simulink library "NeuroMuscularLibrary"  (R2019a)
settings: Solver=ode45  StartTime=0.0  StopTime=10.0  RelTol=1e-3  EnableMultiTasking=on
undefined symbols (not defined in the file): a2loptHAB, a2loptHAD, a2loptHAMsw, a2loptRFsw, ankle_height, aRefHAB, aRefHAD, aRefHAMsw, aRefRFsw, c, c_jointstop, deltaLegAngleThr, DeltaThRef, eref, Fmax, FmaxGLU, footBallToAnkleDist, footBallToCGDist, footBallToCGDist_y, footBallToHeelDist, footCenterlineToBall, footCenterlineToHeel, footInertia, footLength, footMass, FT, FT_GLU, GainDphiHATGLUst, GainDphiHATHABst, GainDphiHATHADst, GainDphiHATHFLst, GainFGASst, GainFGLUst, GainFHABst, GainFHAMst, GainFSOLst, GainFSOLTAst, GainFVASst, GainLBFSHst, GainLBFSHVASst, GainLGLUsw, GainLHABsw, GainLHADsw, GainLHAMGLUsw, GainLHAMsw, GainLRFHFLsw, GainLTAst, GainLTAsw, GainLVASsw, GainPhiHATGLUst, GainPhiHATHABst, GainPhiHATHADst, GainPhiHATHFLst, GainSGLUcHFLst, GainSGLUHAMst, GainSHABcHABst, GainSHADcHADst, GainSHAMBFSHsw, GainSHAMcHFLst, GainSHAMGASsw ... (+175)
libraries: sm_lib x54, $bdroot x45, nesl_utility x39, simulink x24, simulink_extras x6, vrlib x5, dspsigops x4
(part 2 of 5)

== system NeuroMuscularLibrary/Ground Contact Model 3D ==
  note: 3D Ground Interaction Model
  Env : Inport
  " contact sensor" : simulink/Logic and Bit Operations/Compare To Zero  relop=<=  OutDataTypeStr=boolean
  3D Contact : Subsystem
  Demux : Demux  Outputs=3
  Demux2 : Demux  Outputs=6
  Demux3 : Demux  Outputs=[1 3 3]
  External Force and Torque : sm_lib/Forces and Torques/External Force and Torque  ForceResolutionFrame=World  EnableForceX=on  EnableForceY=on  EnableForceZ=on  EnableForce=off  TorqueResolutionFrame=AttachedFrame  EnableTorqueX=off  EnableTorqueY=off  EnableTorqueZ=off  EnableTorque=off
  Mux1 : Mux  Inputs=3
  Mux2 : Mux  Inputs=3
  Position Velocity Sensor : $bdroot/Position Velocity Sensor  SystemSampleTime=-1
  Simulink-PS Converter : nesl_utility/Simulink-PS Converter  PhysicalDomain=network_engine_domain  SubClassName=ps_input  LeftPortType=input  RightPortType=output  PseudoPeriodic=off  Frequencies=[]  NoiseDistribution=none  NoiseParameters=[]  Unit=1  AffineConversion=off  FilteringAndDerivatives=zero  SimscapeFilterOrder=1  InputFilterTimeConstant=0.001  UdotUserProvided=1
  Simulink-PS Converter1 : nesl_utility/Simulink-PS Converter  PhysicalDomain=network_engine_domain  SubClassName=ps_input  LeftPortType=input  RightPortType=output  PseudoPeriodic=off  Frequencies=[]  NoiseDistribution=none  NoiseParameters=[]  Unit=1  AffineConversion=off  FilteringAndDerivatives=zero  SimscapeFilterOrder=1  InputFilterTimeConstant=0.001  UdotUserProvided=1
  Simulink-PS Converter2 : nesl_utility/Simulink-PS Converter  PhysicalDomain=network_engine_domain  SubClassName=ps_input  LeftPortType=input  RightPortType=output  PseudoPeriodic=off  Frequencies=[]  NoiseDistribution=none  NoiseParameters=[]  Unit=1  AffineConversion=off  FilteringAndDerivatives=provide  SimscapeFilterOrder=1  InputFilterTimeConstant=0.001  UdotUserProvided=0
  Sum2 : Sum  Inputs=-+|
  Sum3 : Sum
  Foot : PMIOPort  Side=Left
  Contact? : Outport  VectorParamsAs1DForOutWhenUnconnected=on
  GRF [N N N] : Outport  Port=2  VectorParamsAs1DForOutWhenUnconnected=on
  wires:
  Demux2/1 -> Mux1/1  "x"
  Demux/1 -> Simulink-PS Converter/1
  Mux2/1 -> 3D Contact/4(vVec [m/s m/s m/s])
  Demux2/5 -> Mux2/2  "dy"
  " contact sensor"/1 -> Contact?/1, 3D Contact/Enable
  3D Contact/2(FtVec [N N N]) -> Sum3/2
  Demux/2 -> Simulink-PS Converter1/1
  Demux2/4 -> Mux2/1  "dx"
  3D Contact/1(FnVec [N N N]) -> Sum3/1
  Demux2/2 -> Mux1/2  "y"
  Sum2/1 -> " contact sensor"/1
  Sum3/1 -> Demux/1, GRF [N N N]/1
  Demux2/3 -> Sum2/2, Mux1/3  "z"
  Demux2/6 -> Mux2/3  "dz"
  Demux/3 -> Simulink-PS Converter2/1
  Demux3/3 -> 3D Contact/2(nVec [m m m])  "Normal Vector"
  Mux1/1 -> 3D Contact/3(pVec [m m m])  "pos"
  Demux3/1 -> Sum2/1  "Ground Height"
  Position Velocity Sensor/1 -> Demux2/1
  Env/1 -> Demux3/1
  Demux3/2 -> 3D Contact/1(RefPt [m m m])  "Reference Point"
  connections:
  External Force and Torque/RConn1 -- Foot/RConn1 -- Position Velocity Sensor/LConn1
  External Force and Torque/LConn1 -- Simulink-PS Converter/RConn1
  External Force and Torque/LConn2 -- Simulink-PS Converter1/RConn1
  Simulink-PS Converter2/RConn1 -- External Force and Torque/LConn3

== system NeuroMuscularLibrary/Ground Height Lookup 3D ==
  LHeel+ : Inport
  LHeel- : Inport  Port=2
  LBall+ : Inport  Port=3
  LBall- : Inport  Port=4
  RHeel+ : Inport  Port=5
  RHeel- : Inport  Port=6
  RBall+ : Inport  Port=7
  RBall- : Inport  Port=8
  HATCG : Inport  Port=9
  Env Lookup{,1..8} (9 alike) : $bdroot/Env Lookup  SystemSampleTime=-1  Latency=0  AutoFrameSizeCalculation=off
  Selector : Selector  InputPortWidth=7  IndexOptions=Index vector (dialog)  Indices=[1]  OutputSizes=1
  Selector1 : Selector  InputPortWidth=6  IndexOptions=Index vector (dialog)  Indices=[1 2 3]  OutputSizes=1
  LHeel+Env : Outport  OutputWhenDisabled=reset  InitialOutput=0  VectorParamsAs1DForOutWhenUnconnected=on
  LHeel-Env : Outport  Port=2  OutputWhenDisabled=reset  InitialOutput=0  VectorParamsAs1DForOutWhenUnconnected=on
  LBallEnv : Outport  Port=3  OutputWhenDisabled=reset  InitialOutput=0  VectorParamsAs1DForOutWhenUnconnected=on
  LBall-Env : Outport  Port=4  OutputWhenDisabled=reset  InitialOutput=0  VectorParamsAs1DForOutWhenUnconnected=on
  RHeel+Env : Outport  Port=5  OutputWhenDisabled=reset  InitialOutput=0  VectorParamsAs1DForOutWhenUnconnected=on
  RHeel-Env : Outport  Port=6  OutputWhenDisabled=reset  InitialOutput=0  VectorParamsAs1DForOutWhenUnconnected=on
  RBall+Env : Outport  Port=7  OutputWhenDisabled=reset  InitialOutput=0  VectorParamsAs1DForOutWhenUnconnected=on
  RBall-Env : Outport  Port=8  OutputWhenDisabled=reset  InitialOutput=0  VectorParamsAs1DForOutWhenUnconnected=on
  "HATGroundz " : Outport  Port=9  OutputWhenDisabled=reset  InitialOutput=0  VectorParamsAs1DForOutWhenUnconnected=on
  wires:
  Selector/1 -> "HATGroundz "/1
  Env Lookup8/1 -> Selector/1
  HATCG/1 -> Selector1/1
  Env Lookup6/1 -> RBall+Env/1
  Env Lookup4/1 -> RHeel+Env/1
  RBall+/1 -> Env Lookup6/1
  RHeel+/1 -> Env Lookup4/1
  Env Lookup2/1 -> LBallEnv/1
  LBall+/1 -> Env Lookup2/1
  Env Lookup/1 -> LHeel+Env/1
  LHeel+/1 -> Env Lookup/1
  LHeel-/1 -> Env Lookup1/1
  Env Lookup1/1 -> LHeel-Env/1
  LBall-/1 -> Env Lookup3/1
  Env Lookup3/1 -> LBall-Env/1
  RHeel-/1 -> Env Lookup5/1
  Env Lookup5/1 -> RHeel-Env/1
  RBall-/1 -> Env Lookup7/1
  Env Lookup7/1 -> RBall-Env/1
  Selector1/1 -> Env Lookup8/1

== system NeuroMuscularLibrary/HAB Link ==
  note: HAB Attachment
  Hip roll angle [rad] : Inport
  Constant : Constant  Value=lslackHAB+loptHAB
  Constant1 : Constant  Value=rHAB
  Constant2 : Constant  Value=phirefHAB
  Gain2 : Gain  Gain=rhoHAB
  Product : Product  RndMeth=Zero
  Sum2 : Sum  Inputs=|+-
  Sum5 : Sum  Inputs=|+-
  lmtu [m] : Outport  VectorParamsAs1DForOutWhenUnconnected=on
  lever [m] : Outport  Port=2  VectorParamsAs1DForOutWhenUnconnected=on
  wires:
  Gain2/1 -> Sum5/2
  Constant1/1 -> lever [m]/1, Product/2
  Sum2/1 -> Product/1
  Constant2/1 -> Sum2/2
  Hip roll angle [rad]/1 -> Sum2/1
  Product/1 -> Gain2/1
  Sum5/1 -> lmtu [m]/1
  Constant/1 -> Sum5/1

== system NeuroMuscularLibrary/HAD Link ==
  note: HAD Attachment
  hip roll angle [rad] : Inport
  Constant : Constant  Value=lslackHAD+loptHAD
  Constant1 : Constant  Value=rHAD
  Constant2 : Constant  Value=phirefHAD
  Gain2 : Gain  Gain=rhoHAD
  Product : Product  RndMeth=Zero
  Sum2 : Sum  Inputs=|+-
  Sum5 : Sum  Inputs=|++
  lmtu [m] : Outport  VectorParamsAs1DForOutWhenUnconnected=on
  lever [m] : Outport  Port=2  VectorParamsAs1DForOutWhenUnconnected=on
  wires:
  Constant/1 -> Sum5/1
  Sum5/1 -> lmtu [m]/1
  Product/1 -> Gain2/1
  hip roll angle [rad]/1 -> Sum2/1
  Constant2/1 -> Sum2/2
  Sum2/1 -> Product/1
  Constant1/1 -> Product/2, lever [m]/1
  Gain2/1 -> Sum5/2

== system NeuroMuscularLibrary/HAM Link ==
  note: HAM Attachment
  hip angle : Inport
  knee angle : Inport  Port=2
  Constant1 : Constant  Value=rHAMk
  Constant10 : Constant  Value=phirefHAMh
  Constant2 : Constant  Value=phirefHAMk
  Constant8 : Constant  Value=rHAMh
  Constant9 : Constant  Value=lslackHAM+loptHAM
  Gain1 : Gain  Gain=rhoHAMh
  Gain5 : Gain  Gain=rhoHAMk
  Product1 : Product  RndMeth=Zero
  Product2 : Product  RndMeth=Zero
  Sum1 : Sum  Inputs=|+-
  Sum2 : Sum  Inputs=|+-
  Sum3 : Sum  Inputs=-+-
  lmtu [m] : Outport  VectorParamsAs1DForOutWhenUnconnected=on
  hip lever [m] : Outport  Port=2  VectorParamsAs1DForOutWhenUnconnected=on
  knee lever [m] : Outport  Port=3  VectorParamsAs1DForOutWhenUnconnected=on
  wires:
  Sum1/1 -> Product2/1
  Constant1/1 -> knee lever [m]/1, Product2/2
  Product1/1 -> Gain1/1
  Constant2/1 -> Sum1/2
  Sum3/1 -> lmtu [m]/1
  Gain1/1 -> Sum3/1
  Constant10/1 -> Sum2/2
  Constant8/1 -> hip lever [m]/1, Product1/2
  Constant9/1 -> Sum3/2
  Gain5/1 -> Sum3/3
  Sum2/1 -> Product1/1
  hip angle/1 -> Sum2/1
  knee angle/1 -> Sum1/1
  Product2/1 -> Gain5/1

== system NeuroMuscularLibrary/HAM amp Link ==
  note: HAM Attachment
  hip angle : Inport
  Constant10 : Constant  Value=phirefHAMh
  Constant8 : Constant  Value=rHAMh
  Constant9 : Constant  Value=lslackHAMamp+loptHAMamp
  Gain1 : Gain  Gain=rhoHAMh
  Product1 : Product  RndMeth=Zero
  Sum2 : Sum  Inputs=|+-
  Sum3 : Sum  Inputs=-+
  lmtu [m] : Outport  VectorParamsAs1DForOutWhenUnconnected=on
  hip lever [m] : Outport  Port=2  VectorParamsAs1DForOutWhenUnconnected=on
  wires:
  hip angle/1 -> Sum2/1
  Sum2/1 -> Product1/1
  Constant9/1 -> Sum3/2
  Constant8/1 -> Product1/2, hip lever [m]/1
  Constant10/1 -> Sum2/2
  Gain1/1 -> Sum3/1
  Sum3/1 -> lmtu [m]/1
  Product1/1 -> Gain1/1

== system NeuroMuscularLibrary/HATs ==
  Brick Solid : sm_lib/Body Elements/Solid  InertiaType=CalculateFromGeometry  Mass=0  MassUnits=kg  CenterOfMass=[0 0 0]  CenterOfMassUnits=m  MomentsOfInertia=[1 1 1]  MomentsOfInertiaUnits=kg*m^2  ProductsOfInertia=[0 0 0]  ProductsOfInertiaUnits=kg*m^2  BasedOnType=Mass  Density=0  DensityUnits=kg/m^3  DoExposeReferenceFrame=on  SerializedFrames=<Frames/>  GraphicType=FromGeometry  MarkerShape=Sphere  MarkerSize=10  GraphicVisPropType=SimpleVisualProperties  GraphicDiffuseColor=[0.5 0.5 0.5]  GraphicSpecularColor=[0.5 0.5 0.5 1.0]  GraphicAmbientColor=[0.15 0.15 0.15 1.0]  GraphicEmissiveColor=[0.0 0.0 0.0 1.0]  GraphicShininess=75  GraphicOpacity=1.0  GeometryShape=Brick  RectangleSize=[1 1]  RectangleSizeUnits=m  BrickDimensions=[hatLength hatThickness hatWidth]  BrickDimensionUnits=m  CylinderRadius=1  CylinderRadiusUnits=m  CylinderLength=1  CylinderLengthUnits=m  SphereRadius=1  SphereRadiusUnits=m  EllipsoidRadii=[1 1 1]  EllipsoidRadiiUnits=m  ExtrusionCrossSection=[1 1; -1 1; -1 -1; 1 -1]  ExtrusionCrossSectionUnits=m  ExtrusionLength=1  ExtrusionLengthUnits=m  PolygonNumSides=3  PolygonOuterRadius=1  PolygonOuterRadiusUnits=m  ExtGeomFileType=STEP  ExtGeomFileUnits=m  RevolutionCrossSection=[1 1; 1 -1; 2 -1; 2 1]  RevolutionCrossSectionUnits=m  RevolutionExtent=Full  RevolutionAngle=180  RevolutionAngleUnits=deg
  Inertia : sm_lib/Body Elements/Inertia  InertiaType=Custom  Mass=hatMass  MassUnits=kg  CenterOfMass=[0 0 0]  CenterOfMassUnits=m  MomentsOfInertia=hatInertia  MomentsOfInertiaUnits=kg*m^2  ProductsOfInertia=[0 0 0]  ProductsOfInertiaUnits=kg*m^2  GraphicType=None  MarkerShape=Inertia  MarkerSize=20  GraphicVisPropType=SimpleVisualProperties  GraphicDiffuseColor=[0.5 0.5 0.5]  GraphicSpecularColor=[0.5 0.5 0.5 1.0]  GraphicAmbientColor=[0.15 0.15 0.15 1.0]  GraphicEmissiveColor=[0.0 0.0 0.0 1.0]  GraphicShininess=75  GraphicOpacity=1.0
  Rigid Transform : sm_lib/Frames and Transforms/Rigid Transform  TranslationMethod=None  TranslationStandardOffset=0  TranslationLengthUnit=m  TranslationStandardAxis=+Z  TranslationCartesianOffset=[0 0 0]  TranslationROffset=0  TranslationROffsetUnits=m  TranslationZOffset=0  TranslationZOffsetUnits=m  TranslationThetaOffset=0  TranslationThetaOffsetUnits=deg  RotationMethod=AlignedAxes  RotationAngleUnits=deg  RotationStandardAxis=+Z  RotationAngle=0.0  RotationArbitraryAxis=[0 0 1]  FollAlignAxisA=+X  BaseAlignAxisA=-Y  FollAlignAxisB=+Z  BaseAlignAxisB=+X  RotationSequenceAxes=FollowerAxes  RotationSequence=XYX  RotationSequenceAngles=[0 0 0]  RotationSequenceAnglesUnits=deg  RotationMatrix=[1 0 0; 0 1 0; 0 0 1]
  To CG : sm_lib/Frames and Transforms/Rigid Transform  TranslationMethod=Cartesian  TranslationStandardOffset=0  TranslationLengthUnit=m  TranslationStandardAxis=+Z  TranslationCartesianOffset=[hatLeftHipToCG 0 hatLeftHipToCenterDistWidth]  TranslationROffset=0  TranslationROffsetUnits=m  TranslationZOffset=0  TranslationZOffsetUnits=m  TranslationThetaOffset=0  TranslationThetaOffsetUnits=deg  RotationMethod=None  RotationAngleUnits=deg  RotationStandardAxis=+Z  RotationAngle=0.0  RotationArbitraryAxis=[0 0 1]  FollAlignAxisA=+X  BaseAlignAxisA=-Y  FollAlignAxisB=+Z  BaseAlignAxisB=+X  RotationSequenceAxes=FollowerAxes  RotationSequence=XYX  RotationSequenceAngles=[0 0 0]  RotationSequenceAnglesUnits=deg  RotationMatrix=[1 0 0; 0 1 0; 0 0 1]
  To center : sm_lib/Frames and Transforms/Rigid Transform  TranslationMethod=Cartesian  TranslationStandardOffset=0  TranslationLengthUnit=m  TranslationStandardAxis=+Z  TranslationCartesianOffset=[hatLength/2 0 hatLeftHipToCenterDistWidth]  TranslationROffset=0  TranslationROffsetUnits=m  TranslationZOffset=0  TranslationZOffsetUnits=m  TranslationThetaOffset=0  TranslationThetaOffsetUnits=deg  RotationMethod=None  RotationAngleUnits=deg  RotationStandardAxis=+Z  RotationAngle=0.0  RotationArbitraryAxis=[0 0 1]  FollAlignAxisA=+Z  BaseAlignAxisA=-X  FollAlignAxisB=+Y  BaseAlignAxisB=+Y  RotationSequenceAxes=FollowerAxes  RotationSequence=XYX  RotationSequenceAngles=[0 0 0]  RotationSequenceAnglesUnits=deg  RotationMatrix=[1 0 0; 0 1 0; 0 0 1]
  To right hip : sm_lib/Frames and Transforms/Rigid Transform  TranslationMethod=Cartesian  TranslationStandardOffset=0  TranslationLengthUnit=m  TranslationStandardAxis=+Z  TranslationCartesianOffset=[-2*hatLeftHipToCenterDistWidth 0 0]  TranslationROffset=0  TranslationROffsetUnits=m  TranslationZOffset=0  TranslationZOffsetUnits=m  TranslationThetaOffset=0  TranslationThetaOffsetUnits=deg  RotationMethod=AlignedAxes  RotationAngleUnits=deg  RotationStandardAxis=+Z  RotationAngle=0.0  RotationArbitraryAxis=[0 0 1]  FollAlignAxisA=+X  BaseAlignAxisA=-Z  FollAlignAxisB=+Y  BaseAlignAxisB=+Y  RotationSequenceAxes=FollowerAxes  RotationSequence=XYX  RotationSequenceAngles=[0 0 0]  RotationSequenceAnglesUnits=deg  RotationMatrix=[1 0 0; 0 1 0; 0 0 1]
  To top : sm_lib/Frames and Transforms/Rigid Transform  TranslationMethod=Cartesian  TranslationStandardOffset=0  TranslationLengthUnit=m  TranslationStandardAxis=+Z  TranslationCartesianOffset=[hatLength 0 hatLeftHipToCenterDistWidth]  TranslationROffset=0  TranslationROffsetUnits=m  TranslationZOffset=0  TranslationZOffsetUnits=m  TranslationThetaOffset=0  TranslationThetaOffsetUnits=deg  RotationMethod=None  RotationAngleUnits=deg  RotationStandardAxis=+Z  RotationAngle=0.0  RotationArbitraryAxis=[0 0 1]  FollAlignAxisA=+X  BaseAlignAxisA=+Y  FollAlignAxisB=+Y  BaseAlignAxisB=+Z  RotationSequenceAxes=FollowerAxes  RotationSequence=XYX  RotationSequenceAngles=[0 0 0]  RotationSequenceAnglesUnits=deg  RotationMatrix=[1 0 0; 0 1 0; 0 0 1]
  "X-medial,  Y-back Z-up, to X-up, Y-back, Z lateral" : sm_lib/Frames and Transforms/Rigid Transform  TranslationMethod=None  TranslationStandardOffset=0  TranslationLengthUnit=m  TranslationStandardAxis=+Z  TranslationCartesianOffset=[0 0 0]  TranslationROffset=0  TranslationROffsetUnits=m  TranslationZOffset=0  TranslationZOffsetUnits=m  TranslationThetaOffset=0  TranslationThetaOffsetUnits=deg  RotationMethod=AlignedAxes  RotationAngleUnits=deg  RotationStandardAxis=+Z  RotationAngle=0.0  RotationArbitraryAxis=[0 0 1]  FollAlignAxisA=+X  BaseAlignAxisA=-Z  FollAlignAxisB=+Y  BaseAlignAxisB=+Y  RotationSequenceAxes=FollowerAxes  RotationSequence=XYX  RotationSequenceAngles=[0 0 0]  RotationSequenceAnglesUnits=deg  RotationMatrix=[1 0 0; 0 1 0; 0 0 1]
  Left hip : PMIOPort  Side=Left
  Right hip : PMIOPort  Port=2  Side=Left
  CG : PMIOPort  Port=3  Side=Right
  Top : PMIOPort  Port=4  Side=Right
  connections:
  To center/LConn1 -- To top/LConn1 -- To right hip/RConn1 -- To CG/LConn1 -- "X-medial,  Y-back Z-up, to X-up, Y-back, Z lateral"/RConn1
  Brick Solid/RConn1 -- To center/RConn1
  To right hip/LConn1 -- Right hip/RConn1
  Left hip/RConn1 -- "X-medial,  Y-back Z-up, to X-up, Y-back, Z lateral"/LConn1
  CG/RConn1 -- Rigid Transform/RConn1 -- Inertia/RConn1
  To CG/RConn1 -- Rigid Transform/LConn1
  Top/RConn1 -- To top/RConn1

== system NeuroMuscularLibrary/HFL Link ==
  note: HFL Attachment
  hip angle [rad] : Inport
  Constant : Constant  Value=lslackHFL+loptHFL
  Constant1 : Constant  Value=rHFL
  Constant2 : Constant  Value=phirefHFL
  Gain2 : Gain  Gain=rhoHFL
  Product : Product  RndMeth=Zero
  Sum2 : Sum  Inputs=|+-
  Sum5 : Sum  Inputs=|++
  lmtu [m] : Outport  VectorParamsAs1DForOutWhenUnconnected=on
  lever [m] : Outport  Port=2  VectorParamsAs1DForOutWhenUnconnected=on
  wires:
  Constant/1 -> Sum5/1
  Sum5/1 -> lmtu [m]/1
  Product/1 -> Gain2/1
  Constant2/1 -> Sum2/2
  Sum2/1 -> Product/1
  Constant1/1 -> Product/2, lever [m]/1
  Gain2/1 -> Sum5/2
  hip angle [rad]/1 -> Sum2/1

== system NeuroMuscularLibrary/Hard Stops ==
  Muscle Torques : Inport
  phiANDdphiHip : Inport  Port=2
  phiANDdphiKnee : Inport  Port=3
  phiANDdphiAnkle : Inport  Port=4
  Muscle Torques R : Inport  Port=5
  phiANDdphiHipR : Inport  Port=6
  Add : Sum
  Add1 : Sum
  Ankle Joint Limit : $bdroot/Overextension//Overflexion Joint Limit  phiUpLimit=phiAnkleUpLimit  phiLowLimit=phiAnkleLowLimit
  Demux{,1..3} (4 alike) : Demux  Outputs=2
  Hip Overextension Joint Limit : $bdroot/Overextension Joint Limit  phiUpLimit=phiHipUpLimit  ext=1
  Hip roll Joint Limit : Subsystem  mask(Overextension/Overflexion Joint Limit){phiUpLimit=phiHipAbdUpLimit, phiLowLimit=phiHipAbdLowLimit}
      mask prompts: phiUpLimit "Upper Limit [rad]"; phiLowLimit "Lower Limit [rad]"
      mask help:
      | This block implents a hard joint limit that will prevent the joint from overextending past the specified upper limit and overflexing below the lower limit.
      |
      | Used for the Ankle Joint.
  Knee Overextension Joint Limit : $bdroot/Overextension Joint Limit  phiUpLimit=phiKneeUpLimit  ext=-1
  Mux : Mux  Inputs=3
  Net Torque : Outport  VectorParamsAs1DForOutWhenUnconnected=on
  Hip Stop Torque : Outport  Port=2  VectorParamsAs1DForOutWhenUnconnected=on
  Knee Stop Torque : Outport  Port=3  VectorParamsAs1DForOutWhenUnconnected=on
  Ankle Stop Torque : Outport  Port=4  VectorParamsAs1DForOutWhenUnconnected=on
  Net Torque R : Outport  Port=5  VectorParamsAs1DForOutWhenUnconnected=on
  Hip R Stop Torque : Outport  Port=6  VectorParamsAs1DForOutWhenUnconnected=on
  wires:
  Knee Overextension Joint Limit/1 -> Knee Stop Torque/1, Mux/2
  Muscle Torques/1 -> Add/1
  Mux/1 -> Add/2
  Ankle Joint Limit/1 -> Ankle Stop Torque/1, Mux/3
  Demux/2 -> Knee Overextension Joint Limit/2
  Demux/1 -> Knee Overextension Joint Limit/1
  Demux1/1 -> Hip Overextension Joint Limit/1
  Demux1/2 -> Hip Overextension Joint Limit/2
  Demux2/1 -> Ankle Joint Limit/1
  Demux2/2 -> Ankle Joint Limit/2
  phiANDdphiKnee/1 -> Demux/1
  Hip Overextension Joint Limit/1 -> Hip Stop Torque/1, Mux/1
  phiANDdphiHip/1 -> Demux1/1
  phiANDdphiAnkle/1 -> Demux2/1
  Add/1 -> Net Torque/1
  Demux3/2 -> Hip roll Joint Limit/2(dphi [rad/s])
  Demux3/1 -> Hip roll Joint Limit/1(phi [rad])
  phiANDdphiHipR/1 -> Demux3/1
  Add1/1 -> Net Torque R/1
  Hip roll Joint Limit/1(M_stop [Nm]) -> Hip R Stop Torque/1, Add1/2
  Muscle Torques R/1 -> Add1/1

== system NeuroMuscularLibrary/Hill Muscle ==
  note: Excitation Contraction Coupling
  note: Muscle-Tendon Dynamics
  STIM : Inport
  lmtc [m] : Inport  Port=2
  1 : Product  Inputs=**  SaturateOnIntegerOverflow=on  InputSameDT=on  OutDataTypeStr=Inherit: Same as first input
  1/lslack : Gain  Gain=1/lslack  SaturateOnIntegerOverflow=on  OutDataTypeStr=Inherit: Same as input  ParamDataTypeStr=Inherit: Same as input
  Add : Sum  Inputs=+-
  BE force-length relation : Subsystem
  CE force-length relation : Subsystem
  CE inverse force-velocity relation : Subsystem
  Constant : Constant  Value=lslack
  ECC TransferFcn : simulink_extras/Additional Linear/Transfer Fcn (with initial outputs)  N=[1]  D="[tau  1]"  Y0=preA  U0=0
      settings: AttributesFormatString=pre-activation: %<Y0>
  Fmax : Gain  Gain=Fmax  SaturateOnIntegerOverflow=on  OutDataTypeStr=Inherit: Same as input  ParamDataTypeStr=Inherit: Same as input
  Fv = Fse / (A*Fce) : Product  Inputs=*/  SaturateOnIntegerOverflow=on  InputSameDT=on  OutDataTypeStr=Inherit: Same as first input
  Integrator : Integrator  InitialConditionSource=external  LowerSaturationLimit=0.05
  PE force-length relation : Subsystem
  SE force-length relation : Subsystem
  Sum : Sum  Inputs=|+-  SaturateOnIntegerOverflow=on  InputSameDT=on  OutDataTypeStr=Inherit: Same as first input
  Sum2 : Sum  Inputs=|-+  SaturateOnIntegerOverflow=on  InputSameDT=on  OutDataTypeStr=Inherit: Same as first input
  Sum3 : Sum  SaturateOnIntegerOverflow=on  InputSameDT=on  OutDataTypeStr=Inherit: Same as first input
  Sum4 : Sum  SaturateOnIntegerOverflow=on  InputSameDT=on  OutDataTypeStr=Inherit: Same as first input
  lce/lopt : Gain  Gain=1/lopt  SaturateOnIntegerOverflow=on  OutDataTypeStr=Inherit: Same as input  ParamDataTypeStr=Inherit: Same as input
  lce/lopt1 : Gain  Gain=1/lopt  SaturateOnIntegerOverflow=on  OutDataTypeStr=Inherit: Same as input  ParamDataTypeStr=Inherit: Same as input
  lopt : Gain  Gain=lopt  SaturateOnIntegerOverflow=on  OutDataTypeStr=Inherit: Same as input  ParamDataTypeStr=Inherit: Same as input
  vmax : Gain  Gain=vmax  SaturateOnIntegerOverflow=on  OutDataTypeStr=Inherit: Same as input  ParamDataTypeStr=Inherit: Same as input
  Fmtc : Outport  InitialOutput=0  VectorParamsAs1DForOutWhenUnconnected=on
  Lce [lopt] : Outport  Port=2  InitialOutput=0  VectorParamsAs1DForOutWhenUnconnected=on
  Vce [lopt] : Outport  Port=3  InitialOutput=0  VectorParamsAs1DForOutWhenUnconnected=on
  Lse : Outport  Port=4  InitialOutput=0  VectorParamsAs1DForOutWhenUnconnected=on
  A : Outport  Port=5  InitialOutput=0  VectorParamsAs1DForOutWhenUnconnected=on
  fce : Outport  Port=6  VectorParamsAs1DForOutWhenUnconnected=on
  wires:
  ECC TransferFcn/1 -> 1/2, A/1
  STIM/1 -> ECC TransferFcn/1
  CE inverse force-velocity relation/1(v[vmax]) -> vmax/1
  Sum3/1 -> Fv = Fse / (A*Fce)/2
  BE force-length relation/1(fbe [Fmax]) -> Sum4/2
  1/1 -> Sum3/2
  PE force-length relation/1(fpe [Fmax]) -> Sum3/1, Add/2
  Sum4/1 -> Add/1, Fv = Fse / (A*Fce)/1  "fse+fbe"
  CE force-length relation/1(fce [Fmax]) -> 1/1  "f_l"
  Constant/1 -> Sum2/1
  Sum2/1 -> Integrator/2
  SE force-length relation/1(fse [Fmax]) -> Sum4/1, Fmax/1
  1/lslack/1 -> SE force-length relation/1(lse [lslack])
  Fmax/1 -> Fmtc/1  "Fmtc"
  lmtc [m]/1 -> Sum/1, Sum2/2  "lmtc"
  vmax/1 -> lopt/1, Vce [lopt]/1  "vce"
  Fv = Fse / (A*Fce)/1 -> CE inverse force-velocity relation/1(Fv[Fmax])  "fv"
  lce/lopt/1 -> PE force-length relation/1(lce [lopt]), BE force-length relation/1(lce [lopt]), CE force-length relation/1(lce [lopt])
  Sum/1 -> Lse/1, 1/lslack/1  "lse"
  Integrator/1 -> lce/lopt1/1, lce/lopt/1, Sum/2  "lce"
  Add/1 -> fce/1
  lce/lopt1/1 -> Lce [lopt]/1
  lopt/1 -> Integrator/1  "vce"

== system NeuroMuscularLibrary/Leg Angle//Length ==
  Constant : Constant  Value=pi
  Demux : Demux  Outputs=2
  Mux : Mux  Inputs=3
  Mux1 : Mux  Inputs=3
  PS-Simulink Converter{,1..6} (7 alike) : nesl_utility/PS-Simulink Converter  PhysicalDomain=network_engine_domain  SubClassName=ps_output  LeftPortType=input  RightPortType=output  PseudoPeriodic=off  Frequencies=[]  Unit=m  AffineConversion=off
  Position Sensor : sm_lib/Frames and Transforms/Transform Sensor  MeasurementFrame=World  SenseAngle=off  SenseAxis=off  SenseAngle1=off  SenseAngle2=off  SenseAngle3=off  SenseQ=off  SenseR=off  SenseOmegaX=off  SenseOmegaY=off  SenseOmegaZ=off  SenseOmega1=off  SenseOmega2=off  SenseOmega3=off  SenseQDot=off  SenseRDot=off  SenseAlphaX=off  SenseAlphaY=off  SenseAlphaZ=off  SenseAlpha1=off  SenseAlpha2=off  SenseAlpha3=off  SenseQDDot=off  SenseRDDot=off  SenseX=on  SenseY=on  SenseZ=on  SenseRad=off  SenseAzim=off  SenseDist=off  SenseInc=off  SenseXDot=off  SenseYDot=off  SenseZDot=off  SenseRadDot=off  SenseAzimDot=off  SenseDistDot=off  SenseIncDot=off  SenseXDDot=off  SenseYDDot=off  SenseZDDot=off  SenseRadDDot=off  SenseAzimDDot=off  SenseDistDDot=off  SenseIncDDot=off
  Position Sensor1 : sm_lib/Frames and Transforms/Transform Sensor  MeasurementFrame=World  SenseAngle=off  SenseAxis=off  SenseAngle1=off  SenseAngle2=off  SenseAngle3=off  SenseQ=off  SenseR=off  SenseOmegaX=off  SenseOmegaY=off  SenseOmegaZ=off  SenseOmega1=off  SenseOmega2=off  SenseOmega3=off  SenseQDot=off  SenseRDot=off  SenseAlphaX=off  SenseAlphaY=off  SenseAlphaZ=off  SenseAlpha1=off  SenseAlpha2=off  SenseAlpha3=off  SenseQDDot=off  SenseRDDot=off  SenseX=on  SenseY=on  SenseZ=on  SenseRad=off  SenseAzim=off  SenseDist=off  SenseInc=off  SenseXDot=off  SenseYDot=off  SenseZDot=off  SenseRadDot=off  SenseAzimDot=off  SenseDistDot=off  SenseIncDot=off  SenseXDDot=off  SenseYDDot=off  SenseZDDot=off  SenseRadDDot=off  SenseAzimDDot=off  SenseDistDDot=off  SenseIncDDot=off
  Selector : Selector  InputPortWidth=3  IndexOptions=Index vector (dialog)  Indices=[3 1]  OutputSizes=1
  Subtract : Sum  Inputs=+-
  Sum : Sum  Inputs=|-+
  Transform Sensor : sm_lib/Frames and Transforms/Transform Sensor  MeasurementFrame=World  SenseAngle=off  SenseAxis=off  SenseAngle1=off  SenseAngle2=off  SenseAngle3=off  SenseQ=off  SenseR=off  SenseOmegaX=off  SenseOmegaY=off  SenseOmegaZ=off  SenseOmega1=off  SenseOmega2=off  SenseOmega3=off  SenseQDot=off  SenseRDot=off  SenseAlphaX=off  SenseAlphaY=off  SenseAlphaZ=off  SenseAlpha1=off  SenseAlpha2=off  SenseAlpha3=off  SenseQDDot=off  SenseRDDot=off  SenseX=off  SenseY=off  SenseZ=off  SenseRad=off  SenseAzim=off  SenseDist=on  SenseInc=off  SenseXDot=off  SenseYDot=off  SenseZDot=off  SenseRadDot=off  SenseAzimDot=off  SenseDistDot=off  SenseIncDot=off  SenseXDDot=off  SenseYDDot=off  SenseZDDot=off  SenseRadDDot=off  SenseAzimDDot=off  SenseDistDDot=off  SenseIncDDot=off
  Trigonometric Function : Trigonometry  Operator=atan2  OutputSignalType=real
  World Frame : sm_lib/Frames and Transforms/World Frame
  Hip : PMIOPort  Side=Left
  Ankle : PMIOPort  Port=2  Side=Left
  Leg Angle : Outport  VectorParamsAs1DForOutWhenUnconnected=on
  Leg Length : Outport  Port=2  VectorParamsAs1DForOutWhenUnconnected=on
  wires:
  PS-Simulink Converter6/1 -> Leg Length/1
  PS-Simulink Converter2/1 -> Mux/3
  PS-Simulink Converter/1 -> Mux/1
  PS-Simulink Converter1/1 -> Mux/2
  PS-Simulink Converter5/1 -> Mux1/3
  PS-Simulink Converter3/1 -> Mux1/1
  PS-Simulink Converter4/1 -> Mux1/2
  Mux/1 -> Subtract/1
  Mux1/1 -> Subtract/2
  Trigonometric Function/1 -> Sum/1
  Sum/1 -> Leg Angle/1
  Constant/1 -> Sum/2
  Subtract/1 -> Selector/1
  Selector/1 -> Demux/1
  Demux/1 -> Trigonometric Function/1
  Demux/2 -> Trigonometric Function/2
  connections:
  PS-Simulink Converter6/LConn1 -- Transform Sensor/RConn2
  PS-Simulink Converter2/LConn1 -- Position Sensor/RConn4
  PS-Simulink Converter/LConn1 -- Position Sensor/RConn2
  Transform Sensor/RConn1 -- Hip/RConn1 -- Position Sensor/RConn1
  PS-Simulink Converter1/LConn1 -- Position Sensor/RConn3
  World Frame/RConn1 -- Position Sensor/LConn1 -- Position Sensor1/LConn1
  PS-Simulink Converter4/LConn1 -- Position Sensor1/RConn3
  PS-Simulink Converter5/LConn1 -- Position Sensor1/RConn4
  PS-Simulink Converter3/LConn1 -- Position Sensor1/RConn2
  Transform Sensor/LConn1 -- Ankle/RConn1 -- Position Sensor1/RConn1

== system NeuroMuscularLibrary/Leg Load ==
  dxThigh [m] : Inport
  FB Gain1 : Gain  Gain=1/DeltaThRef  SaturateOnIntegerOverflow=on  OutDataTypeStr=Inherit: Same as input  ParamDataTypeStr=Inherit: Same as input
  Saturation11 : Saturate  UpperLimit=inf  LowerLimit=0  ZeroCross=off
  smooth2 : TransferFcn  Denominator=[0.02 1]
  LLoad [F] : Outport  VectorParamsAs1DForOutWhenUnconnected=on
  wires:
  Saturation11/1 -> FB Gain1/1
  smooth2/1 -> Saturation11/1
  FB Gain1/1 -> LLoad [F]/1
  dxThigh [m]/1 -> smooth2/1

== system NeuroMuscularLibrary/Leg step length//vel calculator ==
  note: Spatial definitions based on Huxham et al. 2006
  Ankle pos : Inport
  Contralateral ankle pos at initial contact : Inport  Port=2
  Simulation time : Inport  Port=3
  Time of contralateral contact : Inport  Port=4
  Prev step number : Inport  Port=5
  Enable : EnablePort
  Add : Sum
  Add2 : Sum  Inputs=-+
  Add3 : Sum  Inputs=+-
  Add4 : Sum  Inputs=+-
  Constant : Constant
  Delay One Step : Delay  DelayLength=1
  Delay One Step1 : Delay  DelayLength=1
  Difference : simulink/Discrete/Difference  ICPrevInput=0.0  OutMin=[]  OutMax=[]  OutDataType=fixdt(1, 16)  OutScaling=2^-10  DoSatur=off
  Divide : Product  Inputs=*/
  Divide1 : Product  Inputs=*/
  Dot Product : DotProduct  InputSameDT=on  OutDataTypeStr=Inherit: Inherit via internal rule
  Norm2 : $bdroot/Norm  SystemSampleTime=-1  Latency=0  AutoFrameSizeCalculation=off
  Product : Product  Inputs=/*
  Selector : Selector  InputPortWidth=3  IndexOptions=Index vector (dialog)  Indices=[1 2]  OutputSizes=1
  Selector1 : Selector  InputPortWidth=3  IndexOptions=Index vector (dialog)  Indices=[1 2]  OutputSizes=1
  Step length : Outport  OutputWhenDisabled=reset  InitialOutput=[0]  VectorParamsAs1DForOutWhenUnconnected=on
  Step time : Outport  Port=2  OutputWhenDisabled=reset  InitialOutput=[0]  VectorParamsAs1DForOutWhenUnconnected=on
  Step avg velocity : Outport  Port=3  OutputWhenDisabled=reset  InitialOutput=[0]  VectorParamsAs1DForOutWhenUnconnected=on
  Stride length : Outport  Port=4  OutputWhenDisabled=reset  InitialOutput=[0]  VectorParamsAs1DForOutWhenUnconnected=on
  Stride time : Outport  Port=5  OutputWhenDisabled=reset  InitialOutput=[0]  VectorParamsAs1DForOutWhenUnconnected=on
  Stride avg velocity : Outport  Port=6  OutputWhenDisabled=reset  InitialOutput=[0]  VectorParamsAs1DForOutWhenUnconnected=on
  Step number : Outport  Port=7  InitialOutput=[0]  VectorParamsAs1DForOutWhenUnconnected=on
  wires:
  Time of contralateral contact/1 -> Add2/1
  Add2/1 -> Step time/1, Divide/2
  Divide/1 -> Step avg velocity/1
  Prev step number/1 -> Delay One Step/1
  Constant/1 -> Add/2
  Add/1 -> Step number/1
  Delay One Step/1 -> Add/1
  Ankle pos/1 -> Selector/1
  Simulation time/1 -> Add2/2, Difference/1
  Add4/1 -> Dot Product/1, Norm2/1
  Delay One Step1/1 -> Add4/2
  Contralateral ankle pos at initial contact/1 -> Selector1/1
  Add3/1 -> Dot Product/2
  Selector/1 -> Add4/1, Delay One Step1/1, Add3/1
  Selector1/1 -> Add3/2
  Norm2/1 -> Product/1, Divide1/1, Stride length/1  "c"
  Difference/1 -> Divide1/2, Stride time/1
  Divide1/1 -> Stride avg velocity/1
  Dot Product/1 -> Product/2
  Product/1 -> Divide/1, Step length/1

== system NeuroMuscularLibrary/Muscle Energy ==
  Dynamics : Inport
  Stimulation : Inport  Port=2
  Muscle Energy Umberger (2003) : $bdroot/Muscle Energy Umberger (2003)  lopt=lopt  FT=FT  Fmax=Fmax  vmax=vmax
  Muscle Energy Umberger (2003) TG : $bdroot/Muscle Energy Umberger (2003) TG  lopt=lopt  FT=FT  Fmax=Fmax
  Muscle Energy Umberger (2010) : $bdroot/Muscle Energy Umberger (2010)  lopt=lopt  FT=FT  Fmax=Fmax  vmax=vmax
  Muscle Energy Wang (2012) : $bdroot/Muscle Energy Wang (2012)  lopt=lopt  FT=FT  Fmax=Fmax
  Mux : Mux
  Power : Outport  VectorParamsAs1DForOutWhenUnconnected=on
  wires:
  Dynamics/1 -> Muscle Energy Umberger (2010)/1, Muscle Energy Umberger (2003) TG/1, Muscle Energy Umberger (2003)/1, Muscle Energy Wang (2012)/1
  Stimulation/1 -> Muscle Energy Umberger (2003)/2, Muscle Energy Umberger (2003) TG/2, Muscle Energy Wang (2012)/2, Muscle Energy Umberger (2010)/2
  Mux/1 -> Power/1
  Muscle Energy Umberger (2003)/1 -> Mux/1
  Muscle Energy Umberger (2003) TG/1 -> Mux/2
  Muscle Energy Umberger (2010)/1 -> Mux/3
  Muscle Energy Wang (2012)/1 -> Mux/4

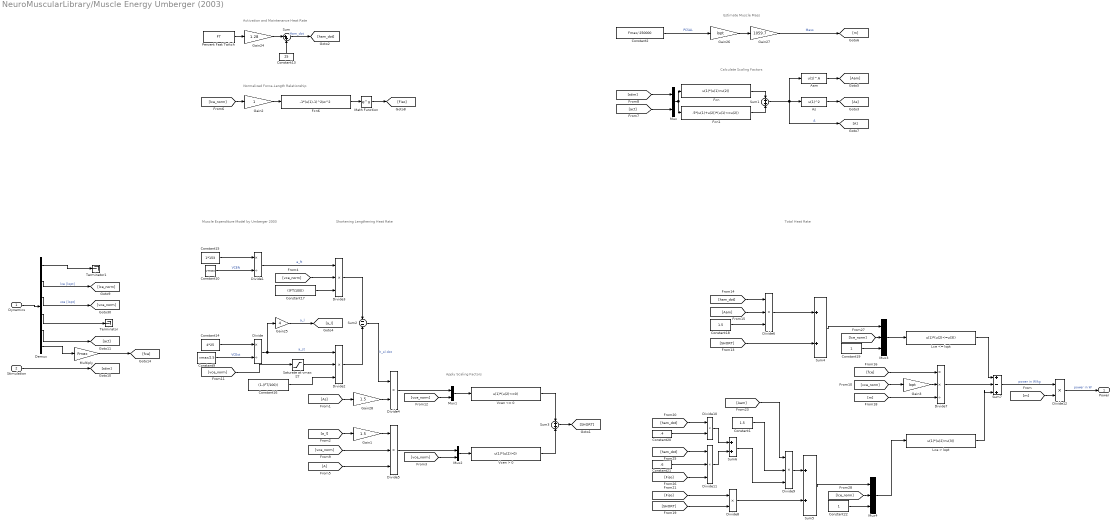
== system NeuroMuscularLibrary/Muscle Energy Umberger (2003) ==
  note: Muscle Expenditure Model by Umberger 2003
  note: Total Heat Rate
  note: Estimate Muscle Mass
  note: Calculate Scaling Factors
  note: Apply Scaling Factors
  note: Shortening Lengthening Heat Rate
  note: Normalized Force-Length Relationship
  note: Activation and Maintenance Heat Rate
  Dynamics : Inport
  Stimulation : Inport  Port=2
  "Aam " : Fcn  Expr=u(1)^.6
  As : Fcn  Expr=u(1)^2
  Constant1 : Constant  Value=1.5
  Constant10 : Constant  Value=vmax
  Constant13 : Constant  Value=25
  Constant14 : Constant  Value=4*25
  Constant15 : Constant  Value=1*153
  Constant16 : Constant  Value=(1-(FT/100))
  Constant17 : Constant  Value=((FT/100))
  Constant18 : Constant  Value=1.5
  Constant19 : Constant
  Constant2 : Constant  Value=Fmax/ 250000
  Constant20 : Constant  Value=.4
  Constant21 : Constant  Value=.6
  Constant22 : Constant
  Constant9 : Constant  Value=vmax/2.5
  Demux : Demux  Outputs=6
  Divide : Product  Inputs=*/
  Divide1 : Product  Inputs=*/
  Divide{4,8,10,12} (4 alike) : Product  Inputs=**
  Divide{2..3,5..6,9,11} (6 alike) : Product  Inputs=***
  Divide7 : Product  Inputs=**/
  Fcn : Fcn  Expr=u(1)*(u(1)>u(2))
  Fcn1 : Fcn  Expr=.5*(u(1)+u(2))*(u(1)<=u(2))
  Fcn6 : Fcn  Expr=-1*(u(1)-1)^2/w^2
  Gain1 : Gain  Gain=1.5
  Gain2 : Gain
  Gain24 : Gain  Gain=1.28
  Gain25 : Gain  Gain=4
  Gain26 : Gain  Gain=lopt
  Gain27 : Gain  Gain=1059.7
  Gain28 : Gain  Gain=1.5
  Gain3 : Gain  Gain=lopt
  Lce <= lopt : Fcn  Expr=u(1)*(u(2)<=u(3))
  Lce > lopt : Fcn  Expr=u(1)*(u(2)>u(3))
  Math Function : Math  SaturateOnIntegerOverflow=on
  Multiply : Gain  Gain=Fmax
  Mux : Mux  Inputs=2
  Mux1 : Mux  Inputs=2
  Mux2 : Mux  Inputs=2
  Mux3 : Mux  Inputs=3
  Mux4 : Mux  Inputs=3
  Percent Fast Twitch : Constant  Value=FT
  Saturate at vmax ST : Saturate  UpperLimit=vmax/2.5  LowerLimit=-vmax/2.5  ZeroCross=off
  Sum : Sum  Inputs=|++
  Sum1 : Sum  Inputs=+|+
  Sum2 : Sum  Inputs=-|-
  Sum3 : Sum  Inputs=+|+
  Sum4 : Sum
  Sum5 : Sum
  Sum6 : Sum
  Sum7 : Sum  Inputs=+-+
  Terminator : Terminator
  Terminator1 : Terminator
  "Vcen <= 0 " : Fcn  Expr=u(1)*(u(2)<=0)
  Vcen > 0 : Fcn  Expr=u(1)*(u(2)>0)
  Power : Outport  VectorParamsAs1DForOutWhenUnconnected=on
  wires:
  Demux/6 -> Multiply/1
  Gain2/1 -> Fcn6/1
  [lce_norm] -> Gain2/1
  Demux/4 -> Terminator/1
  Demux/5 -> [act]
  Demux/3 -> [vce_norm]  "vce [lopt]"
  Demux/2 -> [lce_norm]  "lce [lopt]"
  Demux/1 -> Terminator1/1
  Stimulation/1 -> [stim]
  Dynamics/1 -> Demux/1
  [As] -> Gain28/1
  "Vcen <= 0 "/1 -> Sum3/1
  Sum3/1 -> [SHORT]
  Mux2/1 -> Vcen > 0/1
  Gain27/1 -> [m]  "Mass"
  Constant9/1 -> Divide/2  "VCEst"
  Gain28/1 -> Divide4/2
  [lce_norm] -> Mux3/2
  Mux3/1 -> Lce <= lopt/1
  [SHORT] -> Divide8/2
  Constant2/1 -> Gain26/1  "PCSAL"
  Constant21/1 -> Divide11/2
  [vce_norm] -> Mux2/2
  Percent Fast Twitch/1 -> Gain24/1
  Mux/1 -> Fcn/1, Fcn1/1
  Sum/1 -> [ham_dot]  "Ham_dot"
  Sum2/1 -> Divide4/1  "h_sl dot"
  Constant20/1 -> Divide10/2
  As/1 -> [As]
  Divide8/1 -> Sum5/2
  Constant13/1 -> Sum/2
  Fcn/1 -> Sum1/1
  Fcn1/1 -> Sum1/2
  [vce_norm] -> Divide3/2
  Mux1/1 -> "Vcen <= 0 "/1
  Divide4/1 -> Mux1/1
  Constant15/1 -> Divide1/1
  Constant18/1 -> Divide6/3
  Sum1/1 -> [A], As/1, "Aam "/1  "A"
  [ham_dot] -> Divide6/1
  Divide/1 -> Divide2/1, Gain25/1  "a_st"
  Divide6/1 -> Sum4/1
  Constant14/1 -> Divide/1
  Divide5/1 -> Mux2/1
  Constant22/1 -> Mux4/3
  Vcen > 0/1 -> Sum3/2
  Sum7/1 -> Divide12/1  "power in W/kg"
  [vce_norm] -> Mux1/2
  Divide1/1 -> Divide3/1  "a_ft"
  [vce_norm] -> Saturate at vmax ST/1
  Divide2/1 -> Sum2/2
  Constant10/1 -> Divide1/2  "VCEft"
  "Aam "/1 -> [Aam]
  Math Function/1 -> [Fiso]
  Gain25/1 -> [a_l]  "a_l"
  Divide3/1 -> Sum2/1
  [Fiso] -> Divide11/3
  Constant17/1 -> Divide3/3
  Constant16/1 -> Divide2/3
  Gain1/1 -> Divide5/1
  [Aam] -> Divide6/2
  [a_l] -> Gain1/1
  [vce_norm] -> Divide5/2
  Mux4/1 -> Lce > lopt/1
  Constant19/1 -> Mux3/3
  [SHORT] -> Sum4/2
  Sum6/1 -> Divide9/3
  Sum5/1 -> Mux4/1
  [ham_dot] -> Divide10/1
  [lce_norm] -> Mux4/2
  Divide11/1 -> Sum6/2
  [ham_dot] -> Divide11/1
  [A] -> Divide5/3
  Fcn6/1 -> Math Function/1
  [Fiso] -> Divide8/1
  Divide12/1 -> Power/1  "power in W"
  Sum4/1 -> Mux3/1
  Divide10/1 -> Sum6/1
  Gain24/1 -> Sum/1
  Gain26/1 -> Gain27/1
  [stim] -> Mux/1
  [act] -> Mux/2
  Divide7/1 -> Sum7/2
  [vce_norm] -> Gain3/1
  [fce] -> Divide7/1
  [m] -> Divide7/3
  Constant1/1 -> Divide9/2
  [Aam] -> Divide9/1
  Divide9/1 -> Sum5/1
  [m] -> Divide12/2
  Saturate at vmax ST/1 -> Divide2/2
  Multiply/1 -> [fce]
  Lce <= lopt/1 -> Sum7/1
  Lce > lopt/1 -> Sum7/3
  Gain3/1 -> Divide7/2

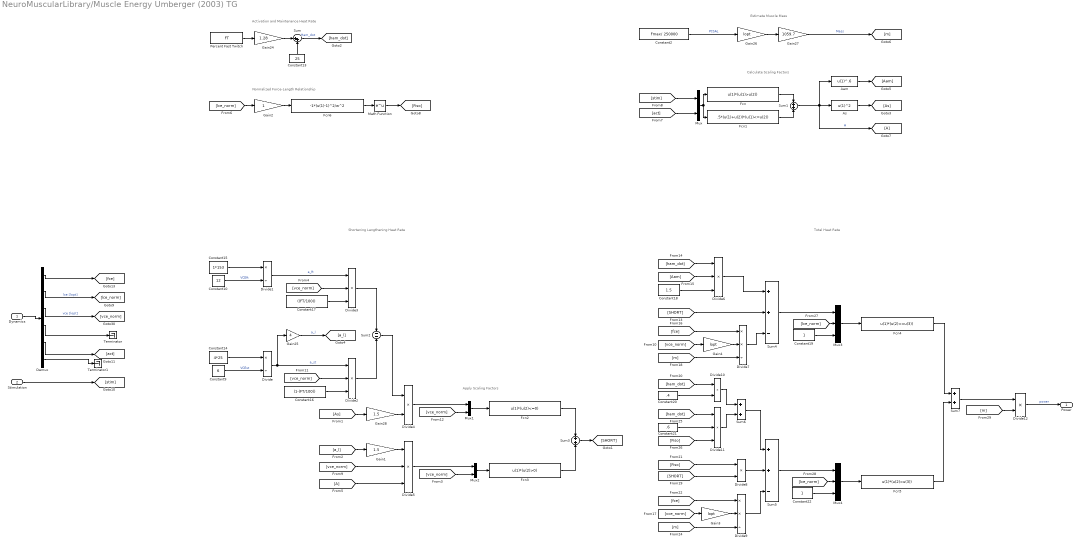
== system NeuroMuscularLibrary/Muscle Energy Umberger (2003) TG ==
  note: Activation and Maintenance Heat Rate
  note: Normalized Force-Length Relationship
  note: Shortening Lengthening Heat Rate
  note: Apply Scaling Factors
  note: Calculate Scaling Factors
  note: Estimate Muscle Mass
  note: Total Heat Rate
  Dynamics : Inport
  Stimulation : Inport  Port=2
  "Aam " : Fcn  Expr=u(1)^.6
  As : Fcn  Expr=u(1)^2
  Constant10 : Constant  Value=12
  Constant13 : Constant  Value=25
  Constant14 : Constant  Value=4*25
  Constant15 : Constant  Value=1*153
  Constant16 : Constant  Value=(1-(FT/100))
  Constant17 : Constant  Value=((FT/100))
  Constant18 : Constant  Value=1.5
  Constant19 : Constant
  Constant2 : Constant  Value=Fmax/ 250000
  Constant20 : Constant  Value=.4
  Constant21 : Constant  Value=.6
  Constant22 : Constant
  Constant9 : Constant  Value=6
  Demux : Demux  Outputs=6
  Divide : Product  Inputs=*/
  Divide1 : Product  Inputs=*/
  Divide{4,8,10,12} (4 alike) : Product  Inputs=**
  Divide{2..3,5..6,11} (5 alike) : Product  Inputs=***
  Divide7 : Product  Inputs=**/
  Divide9 : Product  Inputs=**/
  Fcn : Fcn  Expr=u(1)*(u(1)>u(2))
  Fcn1 : Fcn  Expr=.5*(u(1)+u(2))*(u(1)<=u(2))
  Fcn2 : Fcn  Expr=u(1)*(u(2)<=0)
  Fcn3 : Fcn  Expr=u(1)*(u(2)>0)
  Fcn4 : Fcn  Expr=u(1)*(u(2)<=u(3))
  Fcn5 : Fcn  Expr=u(1)*(u(2)>u(3))
  Fcn6 : Fcn  Expr=-1*(u(1)-1)^2/w^2
  Gain1 : Gain  Gain=1.5
  Gain2 : Gain
  Gain24 : Gain  Gain=1.28
  Gain25 : Gain  Gain=4
  Gain26 : Gain  Gain=lopt
  Gain27 : Gain  Gain=1059.7
  Gain28 : Gain  Gain=1.5
  Gain3 : Gain  Gain=lopt
  Gain4 : Gain  Gain=lopt
  Math Function : Math  SaturateOnIntegerOverflow=on
  Mux : Mux  Inputs=2
  Mux1 : Mux  Inputs=2
  Mux2 : Mux  Inputs=2
  Mux3 : Mux  Inputs=3
  Mux4 : Mux  Inputs=3
  Percent Fast Twitch : Constant  Value=FT
  Sum : Sum  Inputs=|++
  Sum1 : Sum  Inputs=+|+
  Sum2 : Sum  Inputs=-|-
  Sum3 : Sum  Inputs=+|+
  Sum4 : Sum  Inputs=++-
  Sum5 : Sum  Inputs=++-
  Sum6 : Sum
  Sum7 : Sum
  Terminator : Terminator
  Terminator1 : Terminator
  Power : Outport  VectorParamsAs1DForOutWhenUnconnected=on
  wires:
  [m] -> Divide12/2
  [fce] -> Divide7/1
  [act] -> Mux/2
  [stim] -> Mux/1
  Gain26/1 -> Gain27/1
  Gain24/1 -> Sum/1
  Divide10/1 -> Sum6/1
  Divide9/1 -> Sum5/3
  Sum4/1 -> Mux3/1
  Divide12/1 -> Power/1  "power"
  Fcn4/1 -> Sum7/1
  [Fiso] -> Divide8/1
  Fcn6/1 -> Math Function/1
  [A] -> Divide5/3
  [ham_dot] -> Divide11/1
  Divide11/1 -> Sum6/2
  [m] -> Divide9/3
  [lce_norm] -> Mux4/2
  [ham_dot] -> Divide10/1
  Sum5/1 -> Mux4/1
  Sum6/1 -> Sum5/1
  [SHORT] -> Sum4/2
  Constant19/1 -> Mux3/3
  Mux4/1 -> Fcn5/1
  Fcn5/1 -> Sum7/2
  [vce_norm] -> Divide5/2
  [a_l] -> Gain1/1
  [Aam] -> Divide6/2
  Gain1/1 -> Divide5/1
  Constant16/1 -> Divide2/3
  Constant17/1 -> Divide3/3
  [Fiso] -> Divide11/3
  [vce_norm] -> Gain4/1
  Divide3/1 -> Sum2/1
  Gain25/1 -> [a_l]  "a_l"
  Math Function/1 -> [Fiso]
  "Aam "/1 -> [Aam]
  Constant10/1 -> Divide1/2  "VCEft"
  Divide2/1 -> Sum2/2
  [vce_norm] -> Divide2/2
  Divide1/1 -> Divide3/1  "a_ft"
  [vce_norm] -> Mux1/2
  Sum7/1 -> Divide12/1
  Fcn3/1 -> Sum3/2
  Constant22/1 -> Mux4/3
  Divide5/1 -> Mux2/1
  Constant14/1 -> Divide/1
  Divide6/1 -> Sum4/1
  Divide/1 -> Gain25/1, Divide2/1  "a_st"
  [ham_dot] -> Divide6/1
  Sum1/1 -> "Aam "/1, As/1, [A]  "A"
  Constant18/1 -> Divide6/3
  Constant15/1 -> Divide1/1
  Divide4/1 -> Mux1/1
  Mux1/1 -> Fcn2/1
  [vce_norm] -> Divide3/2
  Fcn1/1 -> Sum1/2
  Fcn/1 -> Sum1/1
  [vce_norm] -> Gain3/1
  Divide7/1 -> Sum4/3
  Constant13/1 -> Sum/2
  Divide8/1 -> Sum5/2
  As/1 -> [As]
  Constant20/1 -> Divide10/2
  Sum2/1 -> Divide4/1
  [m] -> Divide7/3
  [fce] -> Divide9/1
  Sum/1 -> [ham_dot]  "Ham_dot"
  Mux/1 -> Fcn1/1, Fcn/1
  Percent Fast Twitch/1 -> Gain24/1
  [vce_norm] -> Mux2/2
  Constant21/1 -> Divide11/2
  Constant2/1 -> Gain26/1  "PCSAL"
  [SHORT] -> Divide8/2
  Mux3/1 -> Fcn4/1
  [lce_norm] -> Mux3/2
  Gain28/1 -> Divide4/2
  Constant9/1 -> Divide/2  "VCEst"
  Gain27/1 -> [m]  "Mass"
  Mux2/1 -> Fcn3/1
  Sum3/1 -> [SHORT]
  Fcn2/1 -> Sum3/1
  [As] -> Gain28/1
  Dynamics/1 -> Demux/1
  Stimulation/1 -> [stim]
  Demux/1 -> [fce]
  Demux/2 -> [lce_norm]  "lce [lopt]"
  Demux/3 -> [vce_norm]  "vce [lopt]"
  Demux/5 -> [act]
  Demux/4 -> Terminator/1
  [lce_norm] -> Gain2/1
  Gain2/1 -> Fcn6/1
  Demux/6 -> Terminator1/1
  Gain3/1 -> Divide9/2
  Gain4/1 -> Divide7/2

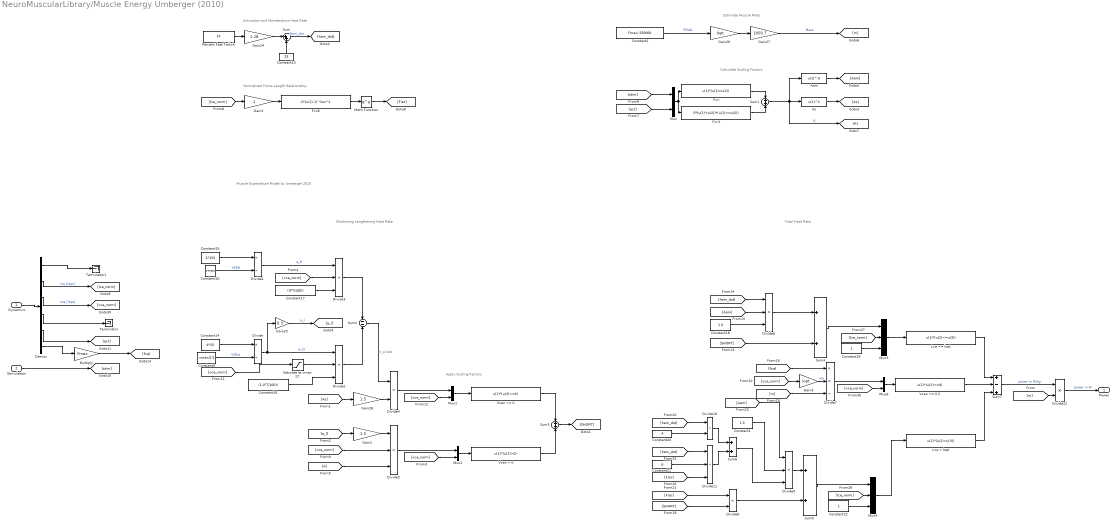
== system NeuroMuscularLibrary/Muscle Energy Umberger (2010) ==
  note: Activation and Maintenance Heat Rate
  note: Normalized Force-Length Relationship
  note: Shortening Lengthening Heat Rate
  note: Apply Scaling Factors
  note: Calculate Scaling Factors
  note: Estimate Muscle Mass
  note: Total Heat Rate
  note: Muscle Expenditure Model by Umberger 2010
  Dynamics : Inport
  Stimulation : Inport  Port=2
  "Aam " : Fcn  Expr=u(1)^.6
  As : Fcn  Expr=u(1)^2
  Constant1 : Constant  Value=1.5
  Constant10 : Constant  Value=vmax
  Constant13 : Constant  Value=25
  Constant14 : Constant  Value=4*25
  Constant15 : Constant  Value=1*153
  Constant16 : Constant  Value=(1-(FT/100))
  Constant17 : Constant  Value=((FT/100))
  Constant18 : Constant  Value=1.5
  Constant19 : Constant
  Constant2 : Constant  Value=Fmax/ 250000
  Constant20 : Constant  Value=.4
  Constant21 : Constant  Value=.6
  Constant22 : Constant
  Constant9 : Constant  Value=vmax/2.5
  Demux : Demux  Outputs=6
  Divide : Product  Inputs=*/
  Divide1 : Product  Inputs=*/
  Divide{4,8,10,12} (4 alike) : Product  Inputs=**
  Divide{2..3,5..6,9,11} (6 alike) : Product  Inputs=***
  Divide7 : Product  Inputs=**/
  Fcn : Fcn  Expr=u(1)*(u(1)>u(2))
  Fcn1 : Fcn  Expr=.5*(u(1)+u(2))*(u(1)<=u(2))
  Fcn6 : Fcn  Expr=-1*(u(1)-1)^2/w^2
  Gain1 : Gain  Gain=1.5
  Gain2 : Gain
  Gain24 : Gain  Gain=1.28
  Gain25 : Gain  Gain=0.3
  Gain26 : Gain  Gain=lopt
  Gain27 : Gain  Gain=1059.7
  Gain28 : Gain  Gain=1.5
  Gain3 : Gain  Gain=lopt
  Lce <= lopt : Fcn  Expr=u(1)*(u(2)<=u(3))
  Lce > lopt : Fcn  Expr=u(1)*(u(2)>u(3))
  Math Function : Math  SaturateOnIntegerOverflow=on
  Multiply : Gain  Gain=Fmax
  Mux{,1..2,6} (4 alike) : Mux  Inputs=2
  Mux3 : Mux  Inputs=3
  Mux4 : Mux  Inputs=3
  Percent Fast Twitch : Constant  Value=FT
  Saturate at vmax ST : Saturate  UpperLimit=vmax/2.5  LowerLimit=-vmax/2.5  ZeroCross=off
  Sum : Sum  Inputs=|++
  Sum1 : Sum  Inputs=+|+
  Sum2 : Sum  Inputs=-|-
  Sum3 : Sum  Inputs=+|+
  Sum4 : Sum
  Sum5 : Sum
  Sum6 : Sum
  Sum7 : Sum  Inputs=+-+
  Terminator : Terminator
  Terminator1 : Terminator
  "Vcen <= 0 " : Fcn  Expr=u(1)*(u(2)<=0)
  Vcen <= 0 2 : Fcn  Expr=u(1)*(u(2)<=0)
  Vcen > 0 : Fcn  Expr=u(1)*(u(2)>0)
  Power : Outport  VectorParamsAs1DForOutWhenUnconnected=on
  wires:
  Lce > lopt/1 -> Sum7/3
  Lce <= lopt/1 -> Sum7/1
  Multiply/1 -> [fce]
  Saturate at vmax ST/1 -> Divide2/2
  [m] -> Divide12/2
  Divide9/1 -> Sum5/1
  [Aam] -> Divide9/1
  Constant1/1 -> Divide9/2
  [m] -> Divide7/3
  [fce] -> Divide7/1
  [vce_norm] -> Gain3/1
  [act] -> Mux/2
  [stim] -> Mux/1
  Gain26/1 -> Gain27/1
  Gain24/1 -> Sum/1
  Divide10/1 -> Sum6/1
  Sum4/1 -> Mux3/1
  Divide12/1 -> Power/1  "power in W"
  [Fiso] -> Divide8/1
  Fcn6/1 -> Math Function/1
  [A] -> Divide5/3
  [ham_dot] -> Divide11/1
  Divide11/1 -> Sum6/2
  [lce_norm] -> Mux4/2
  [ham_dot] -> Divide10/1
  Sum5/1 -> Mux4/1
  Sum6/1 -> Divide9/3
  [SHORT] -> Sum4/2
  Constant19/1 -> Mux3/3
  Mux4/1 -> Lce > lopt/1
  [vce_norm] -> Divide5/2
  [a_l] -> Gain1/1
  [Aam] -> Divide6/2
  Gain1/1 -> Divide5/1
  Constant16/1 -> Divide2/3
  Constant17/1 -> Divide3/3
  [Fiso] -> Divide11/3
  Divide3/1 -> Sum2/1
  Gain25/1 -> [a_l]  "a_l"
  Math Function/1 -> [Fiso]
  "Aam "/1 -> [Aam]
  Constant10/1 -> Divide1/2  "VCEft"
  Divide2/1 -> Sum2/2
  [vce_norm] -> Saturate at vmax ST/1
  Divide1/1 -> Divide3/1  "a_ft"
  [vce_norm] -> Mux1/2
  Sum7/1 -> Divide12/1  "power in W/kg"
  Vcen > 0/1 -> Sum3/2
  Constant22/1 -> Mux4/3
  Divide5/1 -> Mux2/1
  Constant14/1 -> Divide/1
  Divide6/1 -> Sum4/1
  Divide/1 -> Gain25/1, Divide2/1  "a_st"
  [ham_dot] -> Divide6/1
  Sum1/1 -> "Aam "/1, As/1, [A]  "A"
  Constant18/1 -> Divide6/3
  Constant15/1 -> Divide1/1
  Divide4/1 -> Mux1/1
  Mux1/1 -> "Vcen <= 0 "/1
  [vce_norm] -> Divide3/2
  Fcn1/1 -> Sum1/2
  Fcn/1 -> Sum1/1
  Constant13/1 -> Sum/2
  Divide8/1 -> Sum5/2
  As/1 -> [As]
  Constant20/1 -> Divide10/2
  Sum2/1 -> Divide4/1  "h_sl dot"
  Sum/1 -> [ham_dot]  "Ham_dot"
  Mux/1 -> Fcn1/1, Fcn/1
  Percent Fast Twitch/1 -> Gain24/1
  [vce_norm] -> Mux2/2
  Constant21/1 -> Divide11/2
  Constant2/1 -> Gain26/1  "PCSAL"
  [SHORT] -> Divide8/2
  Mux3/1 -> Lce <= lopt/1
  [lce_norm] -> Mux3/2
  Gain28/1 -> Divide4/2
  Constant9/1 -> Divide/2  "VCEst"
  Gain27/1 -> [m]  "Mass"
  Mux2/1 -> Vcen > 0/1
  Sum3/1 -> [SHORT]
  "Vcen <= 0 "/1 -> Sum3/1
  [As] -> Gain28/1
  Dynamics/1 -> Demux/1
  Stimulation/1 -> [stim]
  Demux/1 -> Terminator1/1
  Demux/2 -> [lce_norm]  "lce [lopt]"
  Demux/3 -> [vce_norm]  "vce [lopt]"
  Demux/5 -> [act]
  Demux/4 -> Terminator/1
  [lce_norm] -> Gain2/1
  Gain2/1 -> Fcn6/1
  Demux/6 -> Multiply/1
  [vce_norm] -> Mux6/2
  Divide7/1 -> Mux6/1
  Mux6/1 -> Vcen <= 0 2/1
  Vcen <= 0 2/1 -> Sum7/2
  Gain3/1 -> Divide7/2  "vce"
